simulink model "Advance_CONTROLLERwithOL"  (Simulink 7.5)
settings: Solver=ode45  StartTime=0.0  StopTime=10.0  RelTol=1e-3
undefined symbols (not defined in the file): ctrller, scenario
settings Model: Creator=sriddle  LastModifiedBy=sriddle

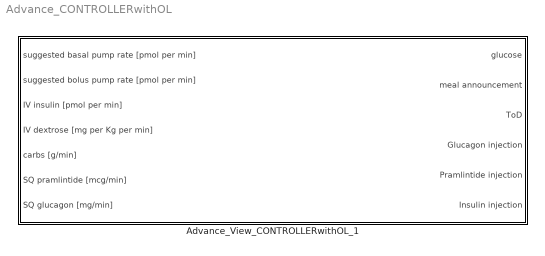
== system Advance_CONTROLLERwithOL ==
  Advance_View_CONTROLLERwithOL_1 : Subsystem

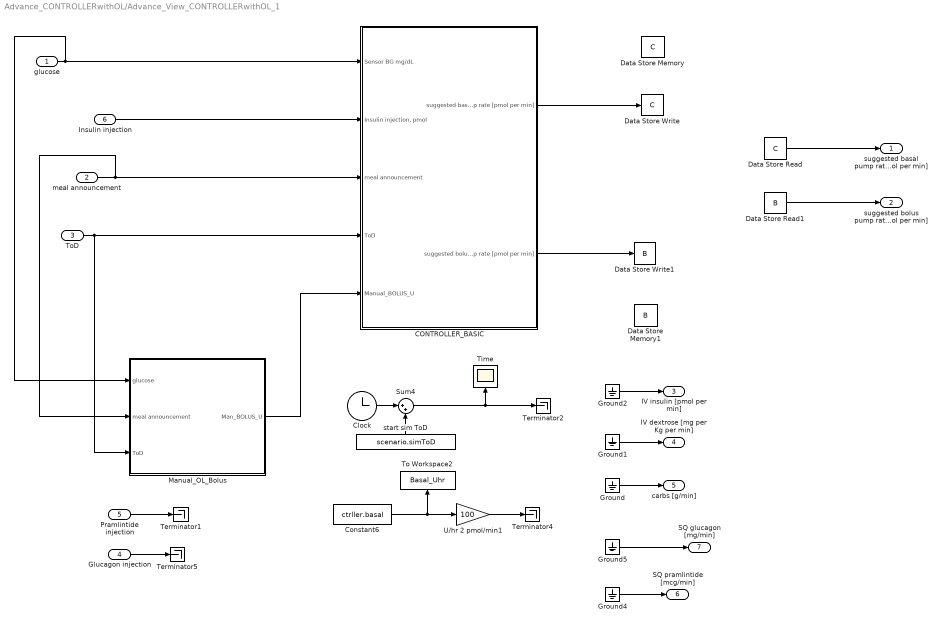
== system Advance_CONTROLLERwithOL/Advance_View_CONTROLLERwithOL_1 ==
  glucose : Inport  OutDataType=sfix(16)  OutScaling=2^0
  meal announcement : Inport  Port=2  OutDataType=sfix(16)  OutScaling=2^0
  ToD : Inport  Port=3  OutDataType=sfix(16)  OutScaling=2^0
  Glucagon injection : Inport  Port=4
  Pramlintide injection : Inport  Port=5
  Insulin injection : Inport  Port=6  OutDataType=sfix(16)  OutScaling=2^0
  CONTROLLER_BASIC : Subsystem  TreatAsAtomicUnit=on
  Clock : Clock
      settings: Decimation=10
  Constant6 : Constant  Value=ctrller.basal
  Data Store Memory : DataStoreMemory  DataStoreName=C  ReadBeforeWriteMsg=warning  WriteAfterWriteMsg=warning  WriteAfterReadMsg=warning  OutDataType=fixdt(1, 16)  OutScaling=2^0
  Data Store Memory1 : DataStoreMemory  DataStoreName=B  ReadBeforeWriteMsg=warning  WriteAfterWriteMsg=warning  WriteAfterReadMsg=warning  OutDataType=fixdt(1, 16)  OutScaling=2^0
  Data Store Read : DataStoreRead  DataStoreName=C  SampleTime=0
  Data Store Read1 : DataStoreRead  DataStoreName=B  SampleTime=0
  Data Store Write : DataStoreWrite  DataStoreName=C  SampleTime=-1
  Data Store Write1 : DataStoreWrite  DataStoreName=B  SampleTime=-1
  Ground{,1..2,4..5} (5 alike) : Ground
  Manual_OL_Bolus : Subsystem
  Sum4 : Sum  Inputs=|++  OutDataType=sfix(16)  OutScaling=2^0
  Terminator{1..2,4..5} (4 alike) : Terminator
  Time : Scope
      settings: YMin=0  YMax=60000  SaveName=ScopeData18
  To Workspace2 : ToWorkspace  VariableName=Basal_Uhr  SampleTime=-1  SaveFormat=Structure
  U/hr 2 pmol/min1 : Gain  Gain=100  ParameterDataType=sfix(16)  ParameterScaling=2^0  OutDataType=sfix(16)  OutScaling=2^0
  start sim ToD : Constant  Value=scenario.simToD  OutDataType=sfix(16)  OutScaling=2^0
  suggested basal pump rate [pmol per min] : Outport  OutDataType=sfix(16)  OutScaling=2^0
  suggested bolus pump rate [pmol per min] : Outport  Port=2  OutDataType=sfix(16)  OutScaling=2^0
  IV insulin [pmol per min] : Outport  Port=3  OutDataType=sfix(16)  OutScaling=2^0
  IV dextrose [mg per Kg per min] : Outport  Port=4  OutDataType=sfix(16)  OutScaling=2^0
  carbs [g/min] : Outport  Port=5  OutDataType=sfix(16)  OutScaling=2^0
  SQ pramlintide [mcg/min] : Outport  Port=6
  SQ glucagon [mg/min] : Outport  Port=7
  wires:
  Ground1/1 -> IV dextrose [mg per Kg per min]/1
  Ground2/1 -> IV insulin [pmol per min]/1
  Ground/1 -> carbs [g/min]/1
  Clock/1 -> Sum4/1
  Sum4/1 -> Terminator2/1, Time/1
  start sim ToD/1 -> Sum4/2
  U/hr 2 pmol/min1/1 -> Terminator4/1
  Constant6/1 -> U/hr 2 pmol/min1/1, To Workspace2/1
  Data Store Read1/1 -> suggested bolus pump rate [pmol per min]/1
  Data Store Read/1 -> suggested basal pump rate [pmol per min]/1
  glucose/1 -> CONTROLLER_BASIC/1(Sensor BG mg/dL), Manual_OL_Bolus/1(glucose)
  Insulin injection/1 -> CONTROLLER_BASIC/2("Insulin injection, pmol")
  meal announcement/1 -> CONTROLLER_BASIC/3(meal announcement), Manual_OL_Bolus/2(meal announcement)
  ToD/1 -> CONTROLLER_BASIC/4(ToD), Manual_OL_Bolus/3(ToD)
  Manual_OL_Bolus/1(Man_BOLUS_U) -> CONTROLLER_BASIC/5(Manual_BOLUS_U)
  CONTROLLER_BASIC/2(suggested bolus pump rate [pmol per min]) -> Data Store Write1/1
  CONTROLLER_BASIC/1(suggested basal pump rate [pmol per min]) -> Data Store Write/1
  Pramlintide injection/1 -> Terminator1/1
  Glucagon injection/1 -> Terminator5/1
  Ground5/1 -> SQ glucagon [mg/min]/1
  Ground4/1 -> SQ pramlintide [mcg/min]/1

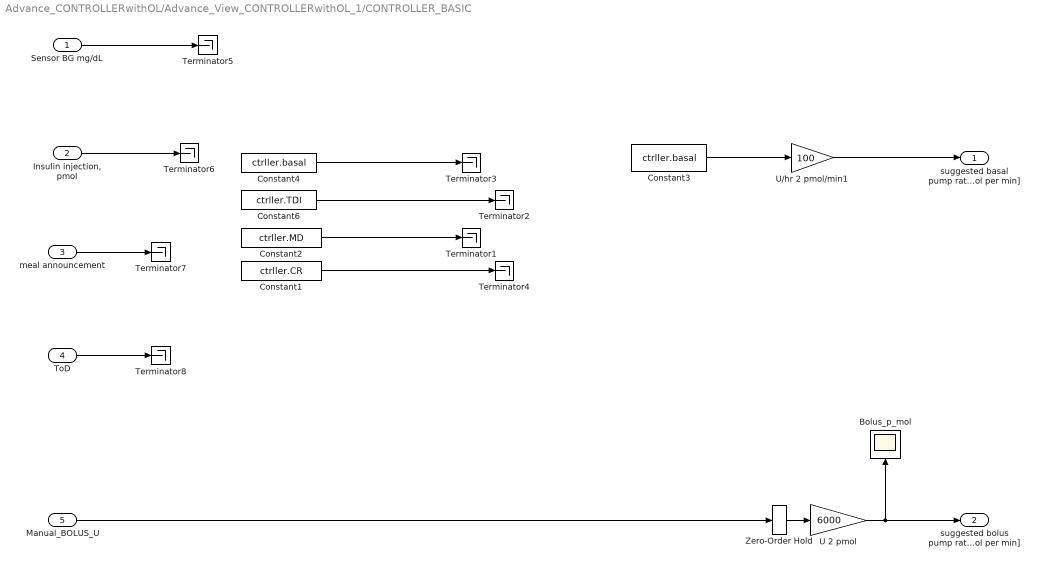
== system Advance_CONTROLLERwithOL/Advance_View_CONTROLLERwithOL_1/CONTROLLER_BASIC ==
  Sensor BG mg/dL : Inport  OutDataType=sfix(16)  OutScaling=2^0
  "Insulin injection, pmol" : Inport  Port=2  OutDataType=sfix(16)  OutScaling=2^0
  meal announcement : Inport  Port=3  OutDataType=sfix(16)  OutScaling=2^0
  ToD : Inport  Port=4  OutDataType=sfix(16)  OutScaling=2^0
  Manual_BOLUS_U : Inport  Port=5  OutDataType=sfix(16)  OutScaling=2^0
  Bolus_p_mol : Scope
      settings: YMin=0  YMax=60000
  Constant1 : Constant  Value=ctrller.CR
  Constant2 : Constant  Value=ctrller.MD
  Constant3 : Constant  Value=ctrller.basal
  Constant4 : Constant  Value=ctrller.basal
  Constant6 : Constant  Value=ctrller.TDI
  Terminator{1..8} (8 alike) : Terminator
  U 2 pmol : Gain  Gain=6000  ParameterDataType=sfix(16)  ParameterScaling=2^0  OutDataType=sfix(16)  OutScaling=2^0
  U/hr 2 pmol/min1 : Gain  Gain=100  ParameterDataType=sfix(16)  ParameterScaling=2^0  OutDataType=sfix(16)  OutScaling=2^0
  Zero-Order Hold : ZeroOrderHold
  suggested basal pump rate [pmol per min] : Outport  OutDataType=sfix(16)  OutScaling=2^0
  suggested bolus pump rate [pmol per min] : Outport  Port=2  OutDataType=sfix(16)  OutScaling=2^0
  wires:
  U 2 pmol/1 -> Bolus_p_mol/1, suggested bolus pump rate [pmol per min]/1
  Zero-Order Hold/1 -> U 2 pmol/1
  Manual_BOLUS_U/1 -> Zero-Order Hold/1
  Constant3/1 -> U/hr 2 pmol/min1/1
  U/hr 2 pmol/min1/1 -> suggested basal pump rate [pmol per min]/1
  Constant1/1 -> Terminator4/1
  Constant4/1 -> Terminator3/1
  Constant6/1 -> Terminator2/1
  Constant2/1 -> Terminator1/1
  Sensor BG mg/dL/1 -> Terminator5/1
  "Insulin injection, pmol"/1 -> Terminator6/1
  meal announcement/1 -> Terminator7/1
  ToD/1 -> Terminator8/1

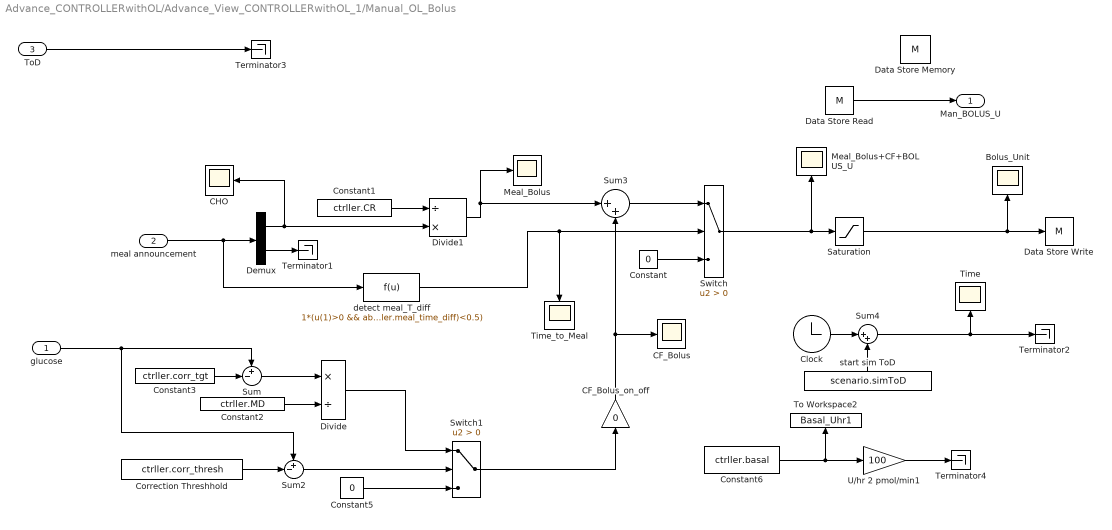
== system Advance_CONTROLLERwithOL/Advance_View_CONTROLLERwithOL_1/Manual_OL_Bolus ==
  glucose : Inport  OutDataType=sfix(16)  OutScaling=2^0
  meal announcement : Inport  Port=2  OutDataType=sfix(16)  OutScaling=2^0
  ToD : Inport  Port=3  OutDataType=sfix(16)  OutScaling=2^0
  Bolus_Unit : Scope
      settings: YMin=0  YMax=60000  SaveName=ScopeData6
  CF_Bolus : Scope
      settings: SaveName=ScopeData7
  CF_Bolus_on_off : Gain  Gain=0  ParameterDataType=fixdt(1, 16)  ParameterScaling=2^0  OutDataType=fixdt(1, 16)  OutScaling=2^0
  CHO : Scope
      settings: YMin=0  YMax=0.01  SaveName=ScopeData8
  Clock : Clock
      settings: Decimation=10
  Constant : Constant  Value=0  OutDataType=sfix(16)  OutScaling=2^0
  Constant1 : Constant  Value=ctrller.CR  OutDataType=sfix(16)  OutScaling=2^0
  Constant2 : Constant  Value=ctrller.MD  OutDataType=sfix(16)  OutScaling=2^0
  Constant3 : Constant  Value=ctrller.corr_tgt  OutDataType=sfix(16)  OutScaling=2^0
  Constant5 : Constant  Value=0  OutDataType=sfix(16)  OutScaling=2^0
  Constant6 : Constant  Value=ctrller.basal
  Correction Threshhold : Constant  Value=ctrller.corr_thresh  OutDataType=sfix(16)  OutScaling=2^0
  Data Store Memory : DataStoreMemory  DataStoreName=M  ReadBeforeWriteMsg=warning  WriteAfterWriteMsg=warning  WriteAfterReadMsg=warning  OutDataType=fixdt(1, 16)  OutScaling=2^0
  Data Store Read : DataStoreRead  DataStoreName=M  SampleTime=0
  Data Store Write : DataStoreWrite  DataStoreName=M  SampleTime=-1
  Demux : Demux  Outputs=2
  Divide : Product  Inputs=*/  OutDataType=sfix(16)  OutScaling=2^-10
  Divide1 : Product  Inputs=/*  OutDataType=sfix(16)  OutScaling=2^-10
  Meal_Bolus : Scope
      settings: SaveName=ScopeData9
  Meal_Bolus+CF+BOLUS_U : Scope
      settings: YMin=0  YMax=3000  SaveName=ScopeData11
  Saturation : Saturate  UpperLimit=100  LowerLimit=0  OutDataType=fixdt(1, 16)  OutScaling=2^0
  Sum : Sum  Inputs=+-|  OutDataType=sfix(16)  OutScaling=2^0
  Sum2 : Sum  Inputs=+-|  OutDataType=sfix(16)  OutScaling=2^0
  Sum3 : Sum  Inputs=|++  OutDataType=sfix(16)  OutScaling=2^0
  Sum4 : Sum  Inputs=|++  OutDataType=sfix(16)  OutScaling=2^0
  Switch : Switch  Criteria=u2 > Threshold  OutDataType=sfix(16)  OutScaling=2^0
  Switch1 : Switch  Criteria=u2 > Threshold  OutDataType=sfix(16)  OutScaling=2^0
  Terminator{1..4} (4 alike) : Terminator
  Time : Scope
      settings: YMin=0  YMax=60000  SaveName=ScopeData12
  Time_to_Meal : Scope
      settings: SaveName=ScopeData13
  To Workspace2 : ToWorkspace  VariableName=Basal_Uhr1  SampleTime=-1  SaveFormat=Structure
  U/hr 2 pmol/min1 : Gain  Gain=100  ParameterDataType=sfix(16)  ParameterScaling=2^0  OutDataType=sfix(16)  OutScaling=2^0
  detect meal_T_diff : Fcn  Expr=1*(u(1)>0 && abs(u(2)+ctrller.meal_time_diff)<0.5)
  start sim ToD : Constant  Value=scenario.simToD  OutDataType=sfix(16)  OutScaling=2^0
  Man_BOLUS_U : Outport  OutDataType=sfix(16)  OutScaling=2^0
  wires:
  Data Store Read/1 -> Man_BOLUS_U/1
  Saturation/1 -> Data Store Write/1, Bolus_Unit/1
  Sum2/1 -> Switch1/2
  Correction Threshhold/1 -> Sum2/2
  Constant5/1 -> Switch1/3
  Constant2/1 -> Divide/2
  Sum/1 -> Divide/1
  Constant3/1 -> Sum/2
  Constant/1 -> Switch/3
  detect meal_T_diff/1 -> Switch/2, Time_to_Meal/1
  ToD/1 -> Terminator3/1
  glucose/1 -> Sum/1, Sum2/1
  Constant1/1 -> Divide1/1
  Demux/1 -> Divide1/2, CHO/1
  meal announcement/1 -> Demux/1, detect meal_T_diff/1
  Demux/2 -> Terminator1/1
  Switch/1 -> Saturation/1, Meal_Bolus+CF+BOLUS_U/1
  Divide1/1 -> Meal_Bolus/1, Sum3/1
  Clock/1 -> Sum4/1
  Sum4/1 -> Terminator2/1, Time/1
  start sim ToD/1 -> Sum4/2
  U/hr 2 pmol/min1/1 -> Terminator4/1
  Constant6/1 -> U/hr 2 pmol/min1/1, To Workspace2/1
  Divide/1 -> Switch1/1
  Switch1/1 -> CF_Bolus_on_off/1
  Sum3/1 -> Switch/1
  CF_Bolus_on_off/1 -> Sum3/2, CF_Bolus/1
